simulink model "silownik_proby"  (R2022a)
settings: Solver=VariableStepAuto  StartTime=0.0  StopTime=10.0  RelTol=1e-3
values from neighbouring files (symbols this model uses):
  A_1 = (pi * (1.2 * 15)^2) / 4 / 10000 * size^2    (= 0.101787601976)    [init.m]    (also in init_notebook.m)
  A_2 = (pi * ((1.2 * 15)^2-(1.2*5)^2)) / 4 / 10000 * size^2    (= 0.0904778684234)    [init.m]    (also in init_notebook.m)
  angles = deg2rad (angles)    [init.m]    (also in init_notebook.m)
  F_force = F_aero.*(0.15 + 0.25 * cord + (x/1000).*cos(angles - beta_angles))/0.225    [init.m]    (also in init_notebook.m)
  K = 1.44 *10^9    (= 1440000000)    [init.m]    (also in init_notebook.m)
  m = 8 * 10^(-6) * pi/4 * (5 * 1.2)^2 * 200 * size^3    (= 0.361911473694)    [init.m]    (also in init_notebook.m)
  V_01 = A_1 * (174 * 1.2/2 - 10 - 5)/100 * size    (= 0.181996232334)    [init.m]    (also in init_notebook.m)
  V_02 = A_2 * (174 * 1.2/2 - 10 - 5)/100 * size    (= 0.161774428741)    [init.m]    (also in init_notebook.m)
  velocity = transpose(velocity)    [init.m]    (also in init_notebook.m)
  x_max = 0.07    [init.m]    (also in init_notebook.m)
  x_min = -0.07    [init.m]    (also in init_notebook.m)
libraries: simulink x1
settings Model: Creator=lukas  LastModifiedBy=lukas

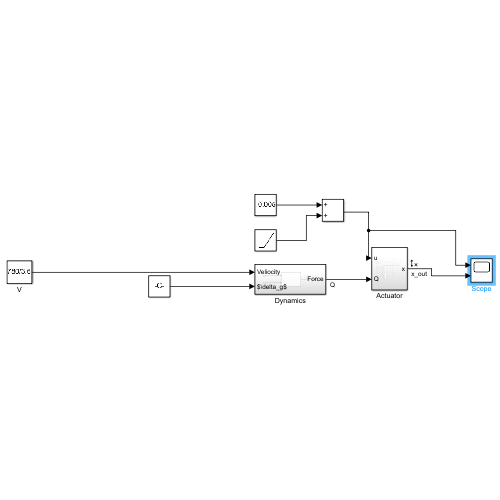
[thumbnail: Simulink's stored preview of the top-level diagram]
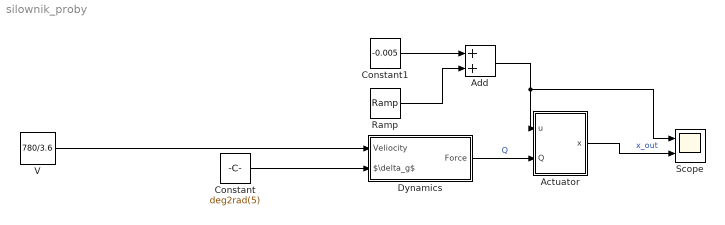
== system silownik_proby ==
  Actuator : Subsystem
  Add : Sum
  Constant : Constant  Value=deg2rad(5)
  Constant1 : Constant  Value=-0.005
  Dynamics : Subsystem
  Ramp : simulink/Sources/Ramp  slope=0.0005  start=0  InitialOutput=0
  Scope : Scope  NumInputPorts=2
  V : Constant  Value=780/3.6
  wires:
  V/1 -> Dynamics/1(Veliocity)
  Dynamics/1(Force) -> Actuator/2(Q)  "Q"
  Constant/1 -> Dynamics/2($\delta_g$)
  Actuator/1(x) -> Scope/2  "x_out"
  Constant1/1 -> Add/1
  Ramp/1 -> Add/2
  Add/1 -> Scope/1, Actuator/1(u)

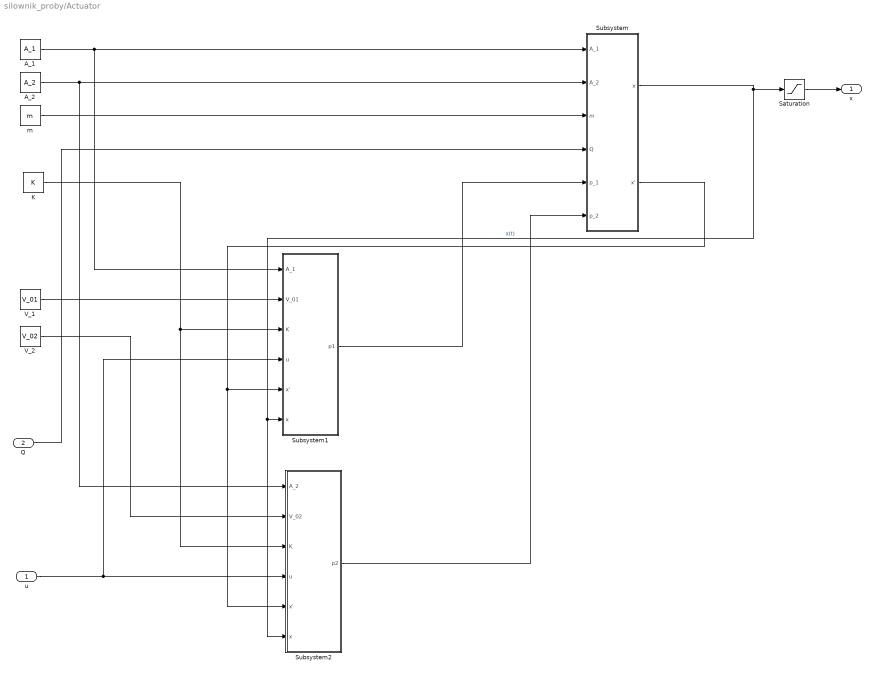
== system silownik_proby/Actuator ==
  u : Inport
  Q : Inport  Port=2
  A_1 : Constant  Value=A_1
  A_2 : Constant  Value=A_2
  K : Constant  Value=K
  Saturation : Saturate  UpperLimit=x_max  LowerLimit=x_min
  Subsystem : Subsystem
  Subsystem1 : Subsystem
  Subsystem2 : Subsystem
  V_1 : Constant  Value=V_01
  V_2 : Constant  Value=V_02
  m : Constant  Value=m
  x : Outport
  wires:
  Subsystem2/1(p2) -> Subsystem/6(p_2)
  V_2/1 -> Subsystem2/2(V_02)
  A_1/1 -> Subsystem1/1(A_1), Subsystem/1(A_1)
  A_2/1 -> Subsystem2/1(A_2), Subsystem/2(A_2)
  Q/1 -> Subsystem/4(Q)
  u/1 -> Subsystem1/4(u), Subsystem2/4(u)
  Subsystem/2(x') -> Subsystem2/5(x'), Subsystem1/5(x')
  K/1 -> Subsystem2/3(K), Subsystem1/3(K)
  Subsystem1/1(p1) -> Subsystem/5(p_1)
  Subsystem/1(x) -> Saturation/1, Subsystem2/6(x), Subsystem1/6(x)  "x(t)"
  V_1/1 -> Subsystem1/2(V_01)
  m/1 -> Subsystem/3(m)
  Saturation/1 -> x/1

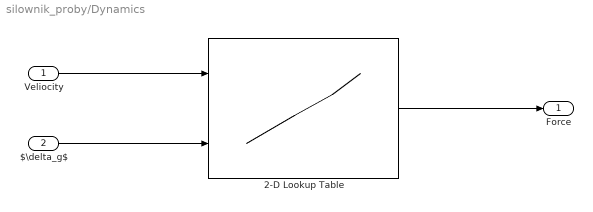
== system silownik_proby/Dynamics ==
  Veliocity : Inport
  $\delta_g$ : Inport  Port=2
  2-D Lookup Table : Lookup_n-D  BreakpointsForDimension1=velocity  BreakpointsForDimension2=angles  Table=F_force  InternalRulePriority=Speed  RndMeth=Simplest
      settings: InputPortMap=u0,u1
  Force : Outport
  wires:
  $\delta_g$/1 -> 2-D Lookup Table/2
  Veliocity/1 -> 2-D Lookup Table/1
  2-D Lookup Table/1 -> Force/1

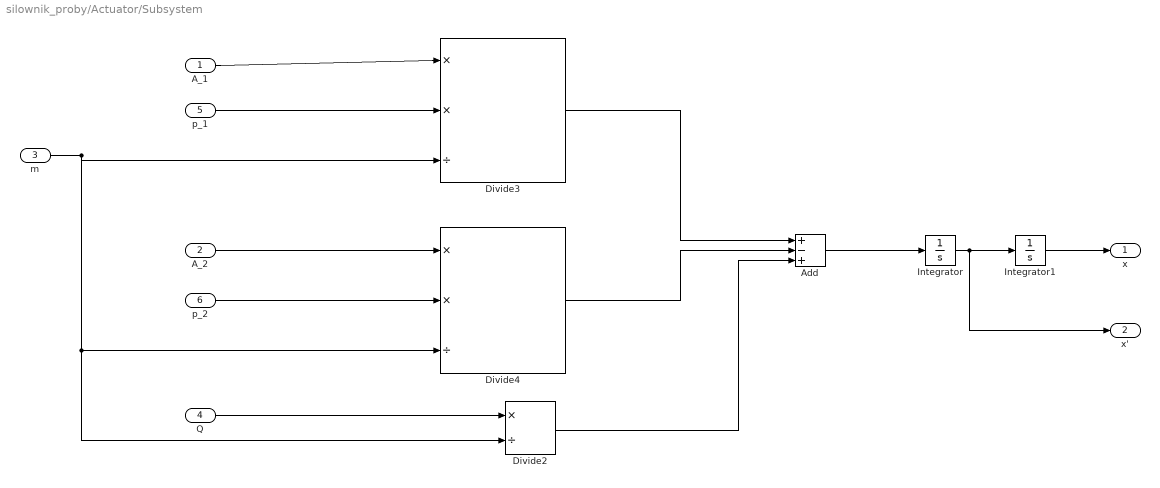
== system silownik_proby/Actuator/Subsystem ==
  A_1 : Inport
  A_2 : Inport  Port=2
  m : Inport  Port=3
  Q : Inport  Port=4
  p_1 : Inport  Port=5
  p_2 : Inport  Port=6
  Add : Sum  Inputs=+-+
  Divide2 : Product  Inputs=*/
  Divide3 : Product  Inputs=**/
  Divide4 : Product  Inputs=**/
  Integrator : Integrator
  Integrator1 : Integrator
  x : Outport
  x' : Outport  Port=2
  wires:
  A_1/1 -> Divide3/1
  p_1/1 -> Divide3/2
  Divide2/1 -> Add/3
  m/1 -> Divide3/3, Divide4/3, Divide2/2
  Q/1 -> Divide2/1
  p_2/1 -> Divide4/2
  A_2/1 -> Divide4/1
  Divide3/1 -> Add/1
  Divide4/1 -> Add/2
  Add/1 -> Integrator/1
  Integrator/1 -> x'/1, Integrator1/1
  Integrator1/1 -> x/1

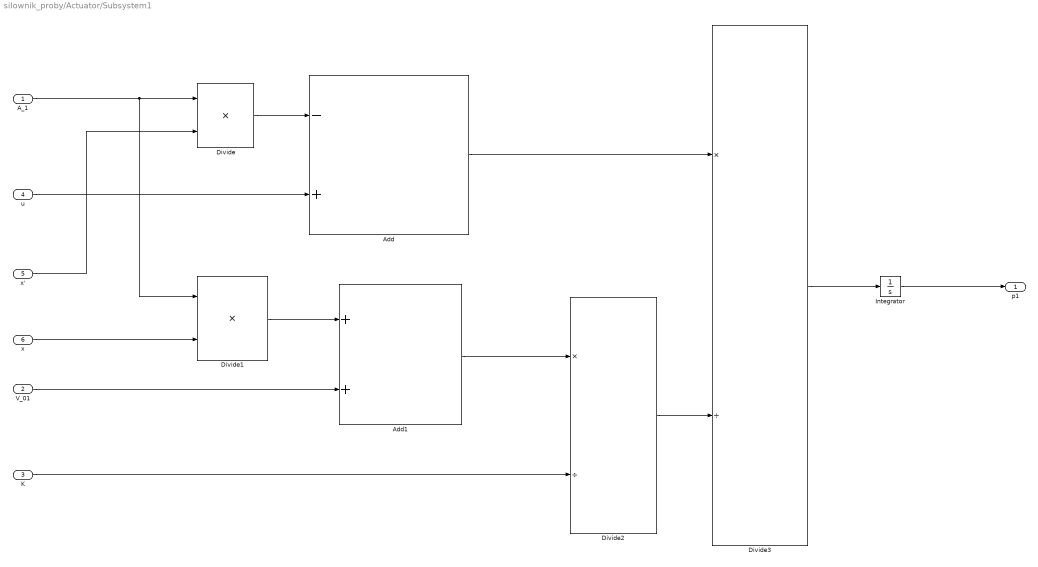
== system silownik_proby/Actuator/Subsystem1 ==
  A_1 : Inport
  V_01 : Inport  Port=2
  K : Inport  Port=3
  u : Inport  Port=4
  x' : Inport  Port=5
  x : Inport  Port=6
  Add : Sum  Inputs=-+
  Add1 : Sum
  Divide : Product  Inputs=**
  Divide1 : Product  Inputs=**
  Divide2 : Product  Inputs=*/
  Divide3 : Product  Inputs=*/
  Integrator : Integrator
  p1 : Outport
  wires:
  A_1/1 -> Divide1/1, Divide/1
  x'/1 -> Divide/2
  Divide/1 -> Add/1
  u/1 -> Add/2
  x/1 -> Divide1/2
  Divide1/1 -> Add1/1
  V_01/1 -> Add1/2
  Add1/1 -> Divide2/1
  K/1 -> Divide2/2
  Add/1 -> Divide3/1
  Divide2/1 -> Divide3/2
  Divide3/1 -> Integrator/1
  Integrator/1 -> p1/1

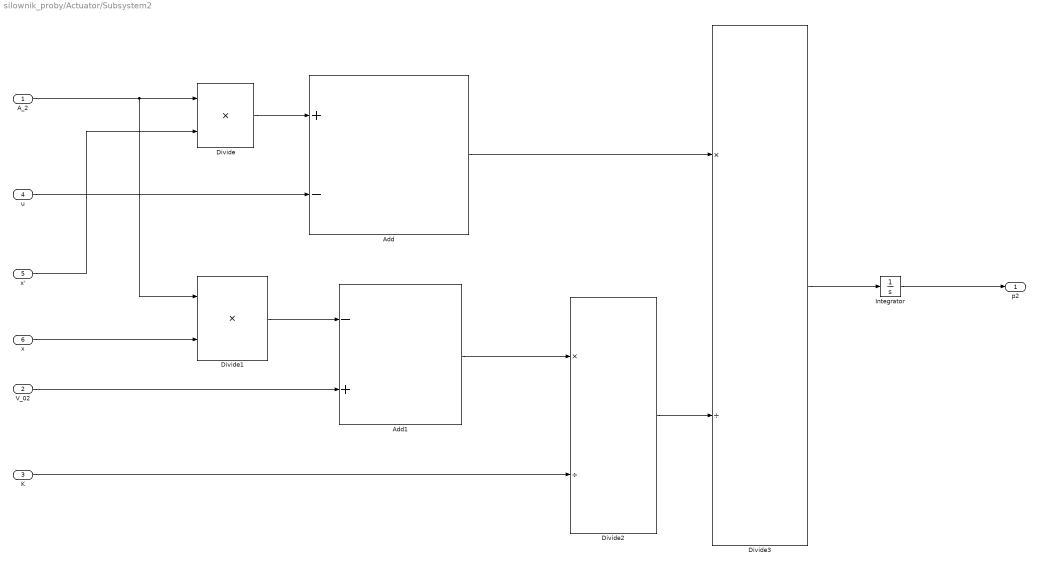
== system silownik_proby/Actuator/Subsystem2 ==
  A_2 : Inport
  V_02 : Inport  Port=2
  K : Inport  Port=3
  u : Inport  Port=4
  x' : Inport  Port=5
  x : Inport  Port=6
  Add : Sum  Inputs=+-
  Add1 : Sum  Inputs=-+
  Divide : Product  Inputs=**
  Divide1 : Product  Inputs=**
  Divide2 : Product  Inputs=*/
  Divide3 : Product  Inputs=*/
  Integrator : Integrator
  p2 : Outport
  wires:
  Integrator/1 -> p2/1
  Divide3/1 -> Integrator/1
  Divide2/1 -> Divide3/2
  Add/1 -> Divide3/1
  K/1 -> Divide2/2
  Add1/1 -> Divide2/1
  V_02/1 -> Add1/2
  Divide1/1 -> Add1/1
  x/1 -> Divide1/2
  u/1 -> Add/2
  Divide/1 -> Add/1
  x'/1 -> Divide/2
  A_2/1 -> Divide/1, Divide1/1
